simulink model "quadcopter_fb_lin_ctrl"  (R2021b)
settings: Solver=FixedStepAuto  StartTime=0.0  StopTime=0.5  FixedStep=0.0001  RelTol=1e-3
values from neighbouring files (symbols this model uses):
  g = 9.81    [quadcopter_dyn_1_param.m]
  kx1 = 10.00    (= 10)    [quadcopter_dyn_1_param.m]
  kx2 = 42.49    [quadcopter_dyn_1_param.m]
  kx3 = 40.27    [quadcopter_dyn_1_param.m]
  kx4 = 13.43    [quadcopter_dyn_1_param.m]
  ky1 = 10.00    (= 10)    [quadcopter_dyn_1_param.m]
  ky2 = 42.49    [quadcopter_dyn_1_param.m]
  ky3 = 40.27    [quadcopter_dyn_1_param.m]
  ky4 = 13.43    [quadcopter_dyn_1_param.m]
  kz1 = 10.00    (= 10)    [quadcopter_dyn_1_param.m]
  kz2 = 42.49    [quadcopter_dyn_1_param.m]
  kz3 = 40.27    [quadcopter_dyn_1_param.m]
  kz4 = 13.43    [quadcopter_dyn_1_param.m]
  l = 1    [quadcopter_dyn_1_param.m]
settings Model: Creator=Chuong  LastModifiedBy=Chuong

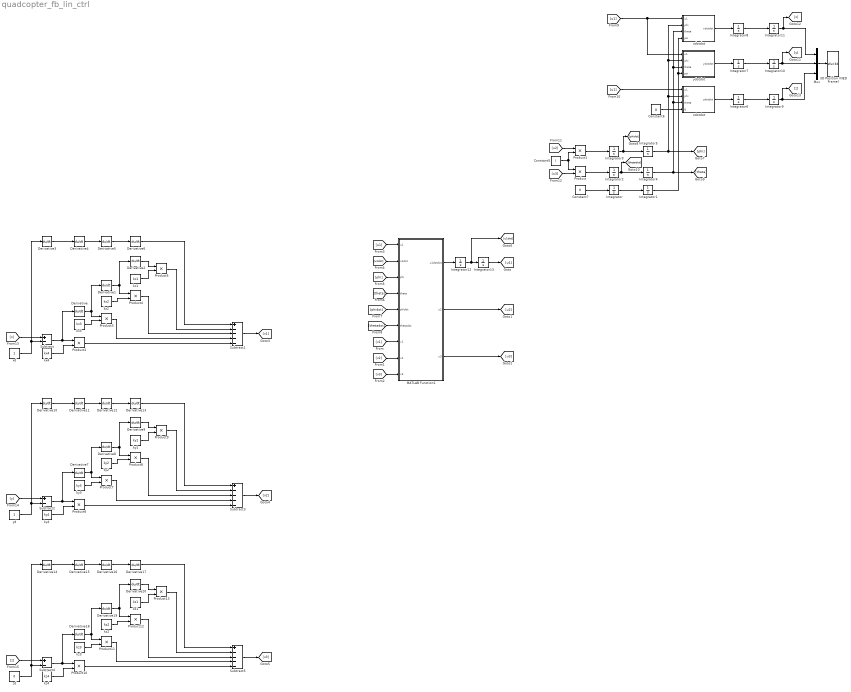
== system quadcopter_fb_lin_ctrl ==
  3D Position (NED Frame) : S-Function  LoadFcn=if exist('sfun3d','file'), sfun3d([],[],[],'LoadBlock'); end  FunctionName=sfun3d  Parameters=ax,T,np,cp,gd,ls,mk,mx,hd,tb  SFunctionDeploymentMode=off  EnableBusSupport=off  mask(3D Graph){np=1, ax=[-10 10 -10 10 -10 10], mx=1e4, T=0.1, cp=[9 6 3], gd=on, hd=off, tb=off, ls=-, mk=none}
      mask prompts: np "Number of moving points (lines)"; ax "Range: [xmin xmax  ymin ymax zmin zmax]"; mx "Max number of points in each line"; T "Sampling Time"; cp "Camera position (use [0 0 1] for 2D XY view)"; gd "Grid (on|off)"; hd "HeadMarkers (on|off)"; tb "Toolbar (on|off)"; ls "LineStyle"; mk "LineMarker"
      mask help:
      | This block plots the position of several points in the XYZ space. The input contains the coordinates of all the points (x1,y1,z1,x2,y2,z2,...).
      | The number of moving points (lines), the XYZ ranges, sampling time, camera position, and grid (among other things) can be set as mask parameters.
      settings: CopyFcn=if exist('sfun3d','file'), sfun3d([],[],[],'CopyBlock'); end  DeleteFcn=if exist('sfun3d','file'), sfun3d([],[],[],'DeleteBlock'); end  NameChangeFcn=if exist('sfun3d','file'), sfun3d([],[],[],'NameChange'); end
      mask Help:
      | This block plots the position of several points in the XYZ space. The input contains the coordinates of all the points (x1,y1,z1,x2,y2,z2,...).
      | The number of moving points (lines), the XYZ ranges, sampling time, camera position, and grid (among other things) can be set as mask parameters.
      mask TypeOptions ls: - | -- | : | -. | none
      mask TypeOptions mk: none | . | + | o | * | x | square | diamond | v | ^ | > | < | pentagram | hexagram
      mask Display: plot([.05 .95 .95 .05 .05],[.45 .45 .95 .95 .45], 0.5+cos(0:0.1:2*pi)*0.3,0.7+sin(0:0.1:2*pi)*0.2)
  Constant5 : Constant  Value=l
  Constant6 : Constant  Value=g
  Constant7 : Constant  Value=0
  Derivative{,1..20} (21 alike) : Derivative
  Integrator{,1..3,6..8,12..13} (9 alike) : Integrator
  Integrator10 : Integrator  InitialCondition=10
  Integrator11 : Integrator  InitialCondition=10
  Integrator4 : Integrator  InitialCondition=0.524
  Integrator5 : Integrator  InitialCondition=0.524
  Integrator9 : Integrator  InitialCondition=20
  MATLAB Function1 : MATLAB Function  TreatAsAtomicUnit=on
  Mux : Mux  Inputs=3
  Product{,1..13} (14 alike) : Product
  Subtract : Sum  Inputs=+-
  Subtract1 : Sum  Inputs=+----
  Subtract2 : Sum  Inputs=+-
  Subtract3 : Sum  Inputs=+----
  Subtract4 : Sum  Inputs=+-
  Subtract5 : Sum  Inputs=+----
  kx1 : Constant  Value=kx1
  kx2 : Constant  Value=kx2
  kx3 : Constant  Value=kx3
  kx4 : Constant  Value=kx4
  ky1 : Constant  Value=ky1
  ky2 : Constant  Value=ky2
  ky3 : Constant  Value=ky3
  ky4 : Constant  Value=ky4
  kz1 : Constant  Value=kz1
  kz2 : Constant  Value=kz2
  kz3 : Constant  Value=kz3
  kz4 : Constant  Value=kz4
  xd : Constant
  xdotdot : MATLAB Function  TreatAsAtomicUnit=on
  yd : Constant
  ydotdot : MATLAB Function  TreatAsAtomicUnit=on
  zd : Constant  Value=0
  zdotdot : MATLAB Function  TreatAsAtomicUnit=on
  wires:
  Integrator/1 -> Integrator1/1
  Product/1 -> Integrator2/1
  Product1/1 -> Integrator3/1
  Integrator2/1 -> [thetadot], Integrator4/1
  Integrator3/1 -> [phidot], Integrator5/1
  Integrator5/1 -> [phi], zdotdot/2(phi), xdotdot/2(phi), ydotdot/2(phi)
  Integrator4/1 -> [theta], xdotdot/3(theta), ydotdot/3(theta), zdotdot/3(theta)
  Integrator1/1 -> xdotdot/4(psi), ydotdot/4(psi)
  Constant6/1 -> zdotdot/4(g)
  zdotdot/1(zdotdot) -> Integrator6/1
  ydotdot/1(ydotdot) -> Integrator7/1
  xdotdot/1(xdotdot) -> Integrator8/1
  Integrator6/1 -> Integrator9/1
  Integrator7/1 -> Integrator10/1
  Integrator8/1 -> Integrator11/1
  Integrator11/1 -> [x], Mux/1
  Integrator10/1 -> [y], Mux/2
  Integrator9/1 -> [z], Mux/3
  Mux/1 -> 3D Position (NED Frame)/1
  MATLAB Function1/1(u1dotdot) -> Integrator12/1
  Integrator12/1 -> [u1dot], Integrator13/1
  Integrator13/1 -> [u1]
  MATLAB Function1/2(u2) -> [u2]
  MATLAB Function1/3(u3) -> [u3]
  [x] -> Subtract/1
  xd/1 -> Derivative3/1, Subtract/2
  Subtract/1 -> Derivative/1, Product2/1
  kx4/1 -> Product2/2
  Product2/1 -> Subtract1/5
  Derivative/1 -> Derivative1/1, Product3/1
  kx3/1 -> Product3/2
  Product3/1 -> Subtract1/4
  Derivative1/1 -> Derivative2/1, Product4/1
  kx2/1 -> Product4/2
  Product4/1 -> Subtract1/3
  kx1/1 -> Product5/2
  Derivative2/1 -> Product5/1
  Product5/1 -> Subtract1/2
  Derivative3/1 -> Derivative4/1
  Derivative4/1 -> Derivative5/1
  Derivative5/1 -> Derivative6/1
  Derivative6/1 -> Subtract1/1
  Subtract1/1 -> [v1]
  [v1] -> MATLAB Function1/7(v1)
  Product9/1 -> Subtract3/2
  Product8/1 -> Subtract3/3
  Subtract2/1 -> Derivative7/1, Product6/1
  Product7/1 -> Subtract3/4
  yd/1 -> Derivative10/1, Subtract2/2
  Derivative9/1 -> Product9/1
  ky4/1 -> Product6/2
  Derivative13/1 -> Subtract3/1
  Derivative11/1 -> Derivative12/1
  ky3/1 -> Product7/2
  Product6/1 -> Subtract3/5
  Derivative10/1 -> Derivative11/1
  ky2/1 -> Product8/2
  Subtract3/1 -> [v2]
  Derivative8/1 -> Derivative9/1, Product8/1
  Derivative12/1 -> Derivative13/1
  ky1/1 -> Product9/2
  [y] -> Subtract2/1
  Derivative7/1 -> Derivative8/1, Product7/1
  [v2] -> MATLAB Function1/8(v2)
  [z] -> Subtract4/1
  Derivative19/1 -> Derivative20/1, Product12/1
  kz2/1 -> Product12/2
  Derivative16/1 -> Derivative17/1
  Subtract5/1 -> [v3]
  Derivative20/1 -> Product13/1
  kz3/1 -> Product11/2
  zd/1 -> Derivative14/1, Subtract4/2
  Derivative17/1 -> Subtract5/1
  Derivative15/1 -> Derivative16/1
  Derivative14/1 -> Derivative15/1
  kz4/1 -> Product10/2
  Product10/1 -> Subtract5/5
  Product12/1 -> Subtract5/3
  kz1/1 -> Product13/2
  Product11/1 -> Subtract5/4
  Derivative18/1 -> Derivative19/1, Product11/1
  Product13/1 -> Subtract5/2
  Subtract4/1 -> Derivative18/1, Product10/1
  [v3] -> MATLAB Function1/9(v3)
  [u1] -> MATLAB Function1/1(u1)
  [u1dot] -> MATLAB Function1/2(u1dot)
  [phi] -> MATLAB Function1/3(phi)
  [theta] -> MATLAB Function1/4(theta)
  [phidot] -> MATLAB Function1/5(phidot)
  [thetadot] -> MATLAB Function1/6(thetadot)
  [u1] -> ydotdot/1(u1), xdotdot/1(u1)
  [u1] -> zdotdot/1(u1)
  Constant7/1 -> Integrator/1
  Constant5/1 -> Product/1, Product1/2
  [u2] -> Product1/1
  [u3] -> Product/2

== matlab function quadcopter_fb_lin_ctrl/xdotdot ==
  data: u1 input; xdotdot output; phi input; theta input; psi input
function xdotdot  = fcn(u1,phi,theta,psi)

xdotdot = u1*(cos(phi)*sin(theta)*cos(psi)+sin(phi)*sin(psi));

== matlab function quadcopter_fb_lin_ctrl/ydotdot ==
  data: u1 input; ydotdot output; phi input; theta input; psi input
function ydotdot = fcn(u1,phi,theta,psi)

ydotdot = u1*(cos(phi)*sin(theta)*sin(psi)-sin(phi)*cos(psi));

== matlab function quadcopter_fb_lin_ctrl/zdotdot ==
  data: u1 input; zdotdot output; phi input; theta input; g input
function zdotdot = fcn(u1,phi,theta,g)

zdotdot = u1*(cos(phi)*cos(theta))-g;

== matlab function quadcopter_fb_lin_ctrl/MATLAB Function1 ==
  data: u1 input; u1dot input; u1dotdot output; phi input; theta input; phidot input; thetadot input; v1 input; u2 output; u3 output; v2 input; v3 input
function [u1dotdot,u2,u3]  = fcn(u1,u1dot,phi,theta,phidot,thetadot,v1,v2,v3)



% u1dotdot = sin(theta)   *(  -2*u1dot*thetadot*cos(theta)    +   u1*(thetadot^2)*sin(theta)  +   v1)...    
%     +   u1*cos(theta)   *(  2*u1dot*phidot*cos(phi)         -   u1*(phidot^2)*sin(phi)      +   v2);
% 
% u2       =  -sin(phi)   *(  -2*u1dot*thetadot*cos(theta)    +   u1*(thetadot^2)*sin(theta)  +   v1)...
%     -   u1*cos(phi)     *(  2*u1dot*thetadot*sin(theta)*cos(phi)    +   2*u1dot*phidot*cos(theta)*sin(phi) ...
%     -   2*u1*thetadot*phidot*sin(theta)*sin(phi)    +   u1*( (thetadot)^2 - (phidot)^2 )*cos(theta)*cos(phi) + v3);
% 
% u3       = cos(theta)*cos(phi)  *(  -2*u1dot*thetadot*cos(theta)    +   u1*(thetadot^2)*sin(theta)  +   v1)...
%     -   u1*sin(theta)*cos(phi)  *(  2*u1dot*phidot*cos(phi)         -   u1*(phidot^2)*sin(phi)      +   v2)...
%     -   u1*cos(theta)*sin(phi)  *(  2*u1dot*thetadot*sin(theta)*cos(phi)    +   2*u1dot*phidot*cos(theta)*sin(phi) ...
%     -   2*u1*thetadot*phidot*sin(theta)*sin(phi)    +   u1*( (thetadot)^2 - (phidot)^2 )*cos(theta)*cos(phi) + v3);

a = [sin(theta)             u1*cos(theta)               0;...
    -sin(phi)               0                           -u1*cos(phi);...
    cos(theta)*cos(phi)     -u1*sin(theta)*cos(phi)     -u1*cos(theta)*sin(phi)];

inv_a = inv(a);

b = [   (  -2*u1dot*thetadot*cos(theta)    +   u1*(thetadot^2)*sin(theta)  +   v1);...
        (  2*u1dot*phidot*cos(phi)         -   u1*(phidot^2)*sin(phi)      +   v2);...
        (  2*u1dot*thetadot*sin(theta)*cos(phi)    +   2*u1dot*phidot*cos(theta)*sin(phi)   -   2*u1*thetadot*phidot*sin(theta)*sin(phi)    +   u1*( (thetadot)^2 - (phidot)^2 )*cos(theta)*cos(phi) + v3)];

c = inv_a*b;

u1dotdot    = c(1);
u2          = c(2);
u3          = c(3);
